simulink model "clark"  (R2022b)
settings: Solver=FixedStepAuto  StartTime=0.0  StopTime=10.0  FixedStep=1e-4  RelTol=1e-3
settings Model: Creator=ssc  LastModifiedBy=ssc

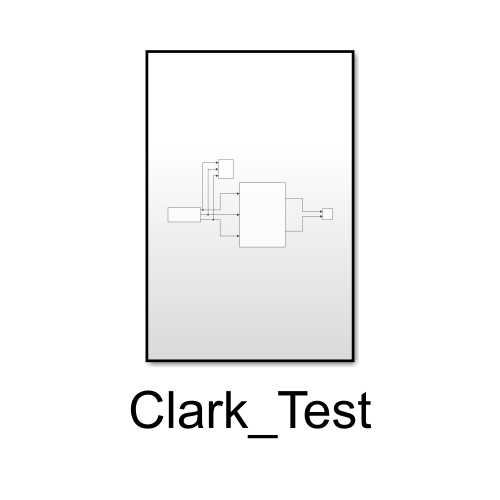
[thumbnail: Simulink's stored preview of the top-level diagram]
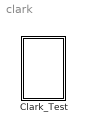
== system clark ==
  Clark_Test : Subsystem

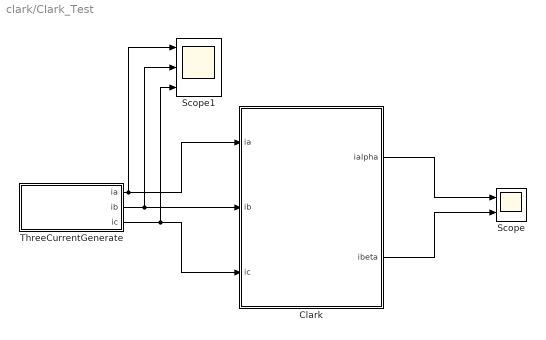
== system clark/Clark_Test ==
  Clark : Subsystem
  Scope : Scope  NumInputPorts=2
  Scope1 : Scope  NumInputPorts=3
  ThreeCurrentGenerate : Subsystem
  wires:
  ThreeCurrentGenerate/3(ic) -> Scope1/3, Clark/3(ic)
  Clark/2(ibeta) -> Scope/2
  ThreeCurrentGenerate/1(ia) -> Scope1/1, Clark/1(ia)
  ThreeCurrentGenerate/2(ib) -> Scope1/2, Clark/2(ib)
  Clark/1(ialpha) -> Scope/1

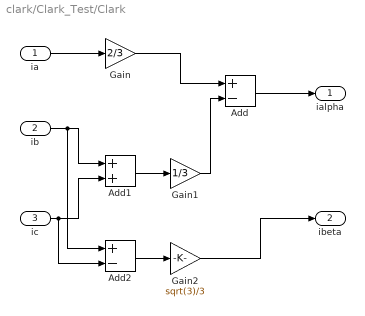
== system clark/Clark_Test/Clark ==
  ia : Inport
  ib : Inport  Port=2
  ic : Inport  Port=3
  Add : Sum  Inputs=+-
  Add1 : Sum
  Add2 : Sum  Inputs=+-
  Gain : Gain  Gain=2/3
  Gain1 : Gain  Gain=1/3
  Gain2 : Gain  Gain=sqrt(3)/3
  ialpha : Outport
  ibeta : Outport  Port=2
  wires:
  ia/1 -> Gain/1
  Gain/1 -> Add/1
  ib/1 -> Add2/1, Add1/1
  Add1/1 -> Gain1/1
  Gain1/1 -> Add/2
  Add/1 -> ialpha/1
  ic/1 -> Add2/2, Add1/2
  Add2/1 -> Gain2/1
  Gain2/1 -> ibeta/1

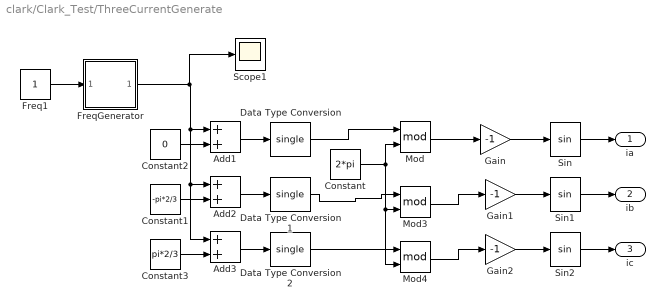
== system clark/Clark_Test/ThreeCurrentGenerate ==
  Add1 : Sum  AccumDataTypeStr=single  OutDataTypeStr=single
  Add2 : Sum  AccumDataTypeStr=single  OutDataTypeStr=single
  Add3 : Sum  AccumDataTypeStr=single  OutDataTypeStr=single
  Constant : Constant  Value=2*pi  OutDataTypeStr=single
  Constant1 : Constant  Value=-pi*2/3  OutDataTypeStr=single
  Constant2 : Constant  Value=0  OutDataTypeStr=single
  Constant3 : Constant  Value=pi*2/3  OutDataTypeStr=single
  Data Type Conversion : DataTypeConversion  OutDataTypeStr=single  SaturateOnIntegerOverflow=off  RndMeth=Floor
  Data Type Conversion1 : DataTypeConversion  OutDataTypeStr=single  SaturateOnIntegerOverflow=off  RndMeth=Floor
  Data Type Conversion2 : DataTypeConversion  OutDataTypeStr=single  SaturateOnIntegerOverflow=off  RndMeth=Floor
  Freq1 : Constant  OutDataTypeStr=single
  FreqGenerator : Subsystem
  Gain : Gain  Gain=-1
  Gain1 : Gain  Gain=-1
  Gain2 : Gain  Gain=-1
  Mod : Math  Operator=mod
  Mod3 : Math  Operator=mod
  Mod4 : Math  Operator=mod
  Scope1 : Scope
  Sin : Trigonometry  ApproximationMethod=Lookup
  Sin1 : Trigonometry  ApproximationMethod=Lookup
  Sin2 : Trigonometry  ApproximationMethod=Lookup
  ia : Outport
  ib : Outport  Port=2
  ic : Outport  Port=3
  wires:
  Gain2/1 -> Sin2/1
  Sin/1 -> ia/1
  Add1/1 -> Data Type Conversion/1
  Gain1/1 -> Sin1/1
  Add2/1 -> Data Type Conversion1/1
  Mod/1 -> Gain/1
  Data Type Conversion/1 -> Mod/1
  Data Type Conversion1/1 -> Mod3/1
  Mod3/1 -> Gain1/1
  Constant/1 -> Mod4/2, Mod3/2, Mod/2
  Freq1/1 -> FreqGenerator/1(Freq)
  Mod4/1 -> Gain2/1
  Add3/1 -> Data Type Conversion2/1
  Sin1/1 -> ib/1
  Gain/1 -> Sin/1
  Constant1/1 -> Add2/2
  Data Type Conversion2/1 -> Mod4/1
  Sin2/1 -> ic/1
  FreqGenerator/1(Theta) -> Scope1/1, Add3/1, Add2/1, Add1/1
  Constant3/1 -> Add3/2
  Constant2/1 -> Add1/2

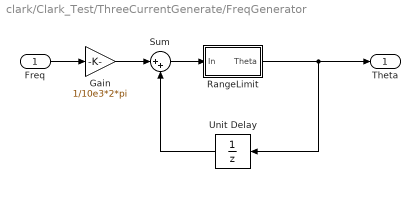
== system clark/Clark_Test/ThreeCurrentGenerate/FreqGenerator ==
  Freq : Inport
  Gain : Gain  Gain=1/10e3*2*pi  OutDataTypeStr=single
  RangeLimit : Subsystem
  Sum : Sum  Inputs=|++  OutDataTypeStr=Inherit: Same as first input
  Unit Delay : UnitDelay  SampleTime=-1  HasFrameUpgradeWarning=on
  Theta : Outport
  wires:
  Freq/1 -> Gain/1
  RangeLimit/1(Theta) -> Theta/1, Unit Delay/1
  Gain/1 -> Sum/1
  Sum/1 -> RangeLimit/1(In)
  Unit Delay/1 -> Sum/2

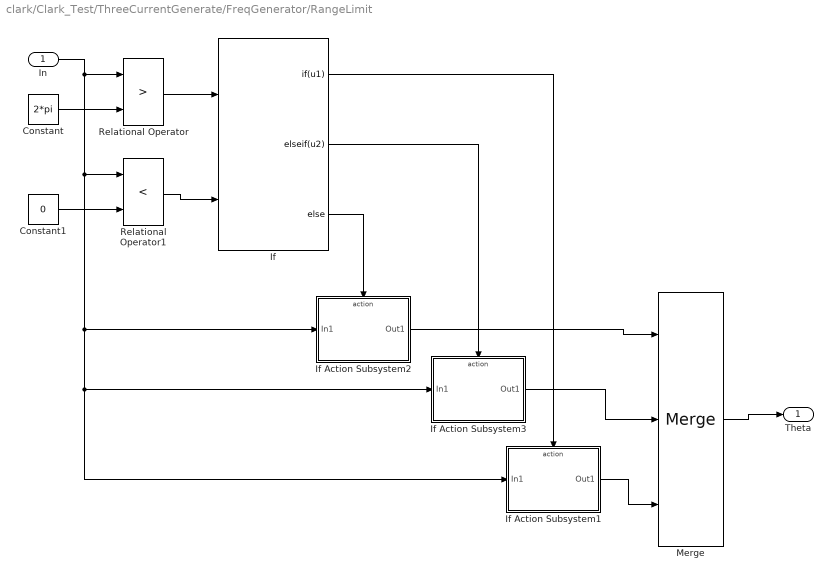
== system clark/Clark_Test/ThreeCurrentGenerate/FreqGenerator/RangeLimit ==
  In : Inport
  Constant : Constant  Value=2*pi  OutDataTypeStr=single  SampleTime=-1
  Constant1 : Constant  Value=0  OutDataTypeStr=single  SampleTime=-1
  If : If  NumInputs=2  IfExpression=u1  ElseIfExpressions=u2
  If Action Subsystem1 : Subsystem  TreatAsAtomicUnit=on
  If Action Subsystem2 : Subsystem  TreatAsAtomicUnit=on
  If Action Subsystem3 : Subsystem  TreatAsAtomicUnit=on
  Merge : Merge  Inputs=3
  Relational Operator : RelationalOperator  Operator=>  OutDataTypeStr=boolean  RndMeth=Simplest  InputSameDT=off
  Relational Operator1 : RelationalOperator  Operator=<  OutDataTypeStr=boolean  RndMeth=Simplest  InputSameDT=off
  Theta : Outport
  wires:
  Relational Operator/1 -> If/1
  Constant/1 -> Relational Operator/2
  In/1 -> Relational Operator1/1, If Action Subsystem2/1(In1), If Action Subsystem3/1(In1), If Action Subsystem1/1(In1), Relational Operator/1
  Merge/1 -> Theta/1
  If/3 -> If Action Subsystem2/Action
  If/1 -> If Action Subsystem1/Action
  If Action Subsystem2/1(Out1) -> Merge/1
  Constant1/1 -> Relational Operator1/2
  Relational Operator1/1 -> If/2
  If/2 -> If Action Subsystem3/Action
  If Action Subsystem1/1(Out1) -> Merge/3
  If Action Subsystem3/1(Out1) -> Merge/2

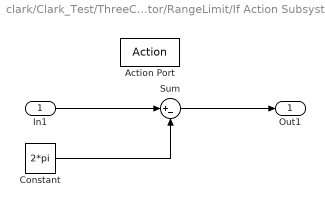
== system clark/Clark_Test/ThreeCurrentGenerate/FreqGenerator/RangeLimit/If Action Subsystem1 ==
  In1 : Inport
  Action Port : ActionPort  ActionPortLabel=if(u1)
  Constant : Constant  Value=2*pi  OutDataTypeStr=single  SampleTime=-1
  Sum : Sum  Inputs=|+-
  Out1 : Outport
  wires:
  In1/1 -> Sum/1
  Constant/1 -> Sum/2
  Sum/1 -> Out1/1

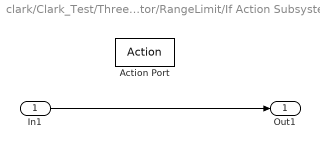
== system clark/Clark_Test/ThreeCurrentGenerate/FreqGenerator/RangeLimit/If Action Subsystem2 ==
  In1 : Inport
  Action Port : ActionPort  ActionPortLabel=else
  Out1 : Outport
  wires:
  In1/1 -> Out1/1

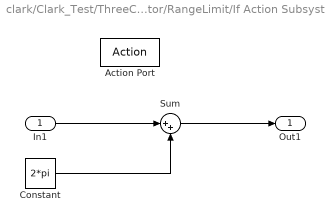
== system clark/Clark_Test/ThreeCurrentGenerate/FreqGenerator/RangeLimit/If Action Subsystem3 ==
  In1 : Inport
  Action Port : ActionPort  ActionPortLabel=elseif(u2)
  Constant : Constant  Value=2*pi  OutDataTypeStr=single  SampleTime=-1
  Sum : Sum  Inputs=|++
  Out1 : Outport
  wires:
  Constant/1 -> Sum/2
  In1/1 -> Sum/1
  Sum/1 -> Out1/1
